simulink model "MotorFramework"  (R2026a)
settings: Solver=FixedStepAuto  StopTime=4  FixedStep=6.25e-5
undefined symbols (not defined in the file): McControl_Params, McRuntime_Init
settings Model: DataDictionary=McData.sldd  Creator=k  LastModifiedBy=k
settings OptimizationCC: UseDivisionForNetSlopeComputation=on  GainParamInheritBuiltInType=on  UseFloatMulNetSlope=on  InlineInvariantSignals=on  NoFixptDivByZeroProtection=on  EfficientFloat2IntCast=on  LifeSpan=1
settings RTWCC: SystemTargetFile=ert.tlc  GenerateReport=on  IncludeHyperlinkInReport=on  GenerateTraceInfo=on  GenerateTraceReport=on  GenerateTraceReportSl=on  GenerateTraceReportSf=on  GenerateTraceReportEml=on  GenerateCodeMetricsReport=on  Description=Embedded Coder
settings ERTTargetCC: GenerateSampleERTMain=on  IncludeMdlTerminateFcn=off  CombineSignalStateStructs=on  SupportComplex=off  SupportContinuousTime=on  SupportNonInlinedSFcns=on

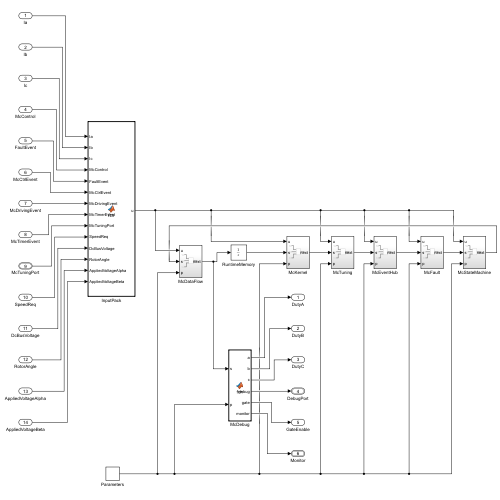
[thumbnail: Simulink's stored preview of the top-level diagram]
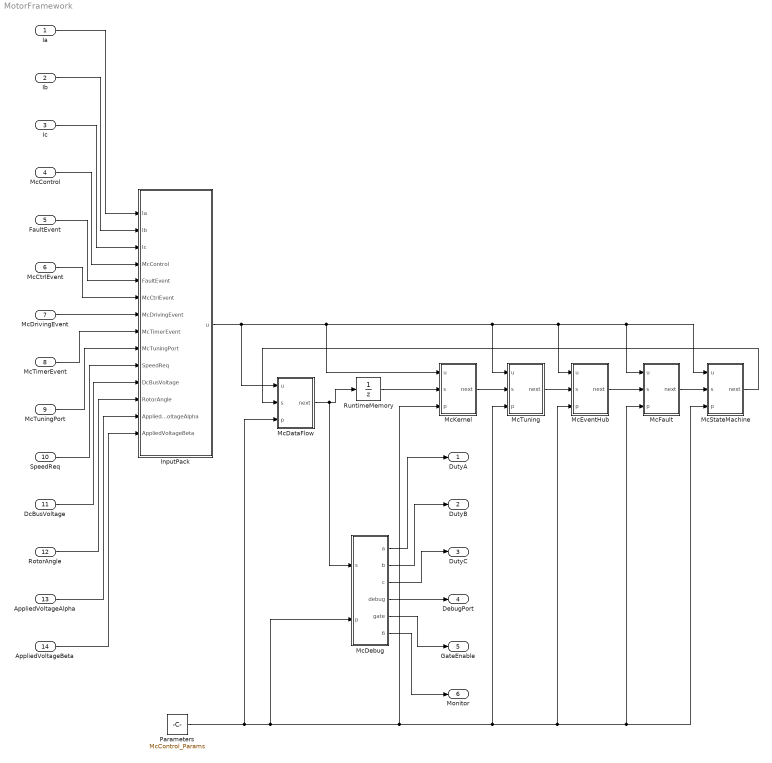
== system MotorFramework ==
  Ia : Inport  OutDataTypeStr=uint16  SampleTime=6.25e-5
  Ib : Inport  Port=2  OutDataTypeStr=uint16  SampleTime=6.25e-5
  Ic : Inport  Port=3  OutDataTypeStr=uint16  SampleTime=6.25e-5
  McControl : Inport  Port=4  OutDataTypeStr=uint8  SampleTime=6.25e-5
  FaultEvent : Inport  Port=5  OutDataTypeStr=boolean  SampleTime=6.25e-5
  McCtrlEvent : Inport  Port=6  OutDataTypeStr=boolean  SampleTime=6.25e-5
  McDrivingEvent : Inport  Port=7  OutDataTypeStr=boolean  SampleTime=6.25e-5
  McTimerEvent : Inport  Port=8  OutDataTypeStr=boolean  SampleTime=6.25e-5
  McTuningPort : Inport  Port=9  OutDataTypeStr=Bus: tMcTuning  SampleTime=6.25e-5
  SpeedReq : Inport  Port=10  OutDataTypeStr=single  SampleTime=6.25e-5
  DcBusVoltage : Inport  Port=11  OutDataTypeStr=single  SampleTime=6.25e-5
  RotorAngle : Inport  Port=12  OutDataTypeStr=single  SampleTime=6.25e-5
  AppliedVoltageAlpha : Inport  Port=13  OutDataTypeStr=single  SampleTime=6.25e-5
  AppliedVoltageBeta : Inport  Port=14  OutDataTypeStr=single  SampleTime=6.25e-5
  InputPack : MATLAB Function  TreatAsAtomicUnit=on
  McDataFlow : Subsystem
  McDebug : MATLAB Function  TreatAsAtomicUnit=on
  McEventHub : Subsystem
  McFault : Subsystem
  McKernel : Subsystem
  McStateMachine : Subsystem
  McTuning : Subsystem
  Parameters : Constant  Value=McControl_Params  OutDataTypeStr=Bus: tMcControlParams
  RuntimeMemory : UnitDelay  InitialCondition=McRuntime_Init  SampleTime=6.25e-5
  DutyA : Outport  OutDataTypeStr=uint16
  DutyB : Outport  Port=2  OutDataTypeStr=uint16
  DutyC : Outport  Port=3  OutDataTypeStr=uint16
  DebugPort : Outport  Port=4  OutDataTypeStr=Bus: tMcDebug
  GateEnable : Outport  Port=5  OutDataTypeStr=boolean
  Monitor : Outport  Port=6  OutDataTypeStr=Bus: tMcMonitor
  wires:
  Ia/1 -> InputPack/1(Ia)
  Ib/1 -> InputPack/2(Ib)
  Ic/1 -> InputPack/3(Ic)
  McControl/1 -> InputPack/4(McControl)
  FaultEvent/1 -> InputPack/5(FaultEvent)
  McCtrlEvent/1 -> InputPack/6(McCtrlEvent)
  McDrivingEvent/1 -> InputPack/7(McDrivingEvent)
  McTimerEvent/1 -> InputPack/8(McTimerEvent)
  McTuningPort/1 -> InputPack/9(McTuningPort)
  SpeedReq/1 -> InputPack/10(SpeedReq)
  DcBusVoltage/1 -> InputPack/11(DcBusVoltage)
  RotorAngle/1 -> InputPack/12(RotorAngle)
  AppliedVoltageAlpha/1 -> InputPack/13(AppliedVoltageAlpha)
  AppliedVoltageBeta/1 -> InputPack/14(AppliedVoltageBeta)
  InputPack/1(u) -> McStateMachine/1(u), McFault/1(u), McEventHub/1(u), McTuning/1(u), McKernel/1(u), McDataFlow/1(u)
  RuntimeMemory/1 -> McKernel/2(s)
  Parameters/1 -> McFault/3(p), McStateMachine/3(p), McEventHub/3(p), McTuning/3(p), McKernel/3(p), McDebug/2(p), McDataFlow/3(p)
  McKernel/1(next) -> McTuning/2(s)
  McTuning/1(next) -> McEventHub/2(s)
  McEventHub/1(next) -> McFault/2(s)
  McFault/1(next) -> McStateMachine/2(s)
  McStateMachine/1(next) -> McDataFlow/2(s)
  McDataFlow/1(next) -> RuntimeMemory/1, McDebug/1(s)
  McDebug/1(a) -> DutyA/1
  McDebug/2(b) -> DutyB/1
  McDebug/3(c) -> DutyC/1
  McDebug/4(debug) -> DebugPort/1
  McDebug/5(gate) -> GateEnable/1
  McDebug/6(monitor) -> Monitor/1

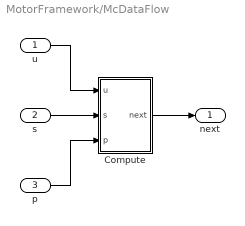
== system MotorFramework/McDataFlow ==
  u : Inport  OutDataTypeStr=Bus: tMcInput  SampleTime=6.25e-5
  s : Inport  Port=2  OutDataTypeStr=Bus: tMcRuntime  SampleTime=6.25e-5
  p : Inport  Port=3  OutDataTypeStr=Bus: tMcControlParams  SampleTime=6.25e-5
  Compute : MATLAB Function  TreatAsAtomicUnit=on
  next : Outport  OutDataTypeStr=Bus: tMcRuntime
  wires:
  Compute/1(next) -> next/1
  p/1 -> Compute/3(p)
  s/1 -> Compute/2(s)
  u/1 -> Compute/1(u)

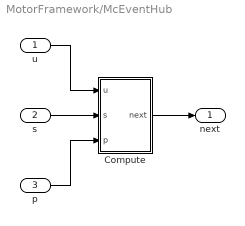
== system MotorFramework/McEventHub ==
  u : Inport  OutDataTypeStr=Bus: tMcInput  SampleTime=6.25e-5
  s : Inport  Port=2  OutDataTypeStr=Bus: tMcRuntime  SampleTime=6.25e-5
  p : Inport  Port=3  OutDataTypeStr=Bus: tMcControlParams  SampleTime=6.25e-5
  Compute : MATLAB Function  TreatAsAtomicUnit=on
  next : Outport  OutDataTypeStr=Bus: tMcRuntime
  wires:
  Compute/1(next) -> next/1
  p/1 -> Compute/3(p)
  s/1 -> Compute/2(s)
  u/1 -> Compute/1(u)

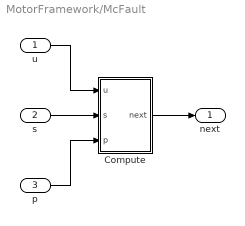
== system MotorFramework/McFault ==
  u : Inport  OutDataTypeStr=Bus: tMcInput  SampleTime=6.25e-5
  s : Inport  Port=2  OutDataTypeStr=Bus: tMcRuntime  SampleTime=6.25e-5
  p : Inport  Port=3  OutDataTypeStr=Bus: tMcControlParams  SampleTime=6.25e-5
  Compute : MATLAB Function  TreatAsAtomicUnit=on
  next : Outport  OutDataTypeStr=Bus: tMcRuntime
  wires:
  Compute/1(next) -> next/1
  p/1 -> Compute/3(p)
  s/1 -> Compute/2(s)
  u/1 -> Compute/1(u)

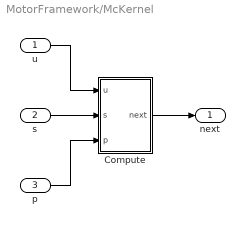
== system MotorFramework/McKernel ==
  u : Inport  OutDataTypeStr=Bus: tMcInput  SampleTime=6.25e-5
  s : Inport  Port=2  OutDataTypeStr=Bus: tMcRuntime  SampleTime=6.25e-5
  p : Inport  Port=3  OutDataTypeStr=Bus: tMcControlParams  SampleTime=6.25e-5
  Compute : MATLAB Function  TreatAsAtomicUnit=on
  next : Outport  OutDataTypeStr=Bus: tMcRuntime
  wires:
  Compute/1(next) -> next/1
  p/1 -> Compute/3(p)
  s/1 -> Compute/2(s)
  u/1 -> Compute/1(u)

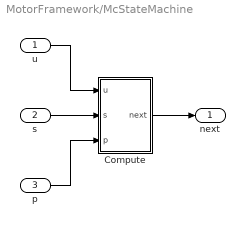
== system MotorFramework/McStateMachine ==
  u : Inport  OutDataTypeStr=Bus: tMcInput  SampleTime=6.25e-5
  s : Inport  Port=2  OutDataTypeStr=Bus: tMcRuntime  SampleTime=6.25e-5
  p : Inport  Port=3  OutDataTypeStr=Bus: tMcControlParams  SampleTime=6.25e-5
  Compute : MATLAB Function  TreatAsAtomicUnit=on
  next : Outport  OutDataTypeStr=Bus: tMcRuntime
  wires:
  Compute/1(next) -> next/1
  p/1 -> Compute/3(p)
  s/1 -> Compute/2(s)
  u/1 -> Compute/1(u)

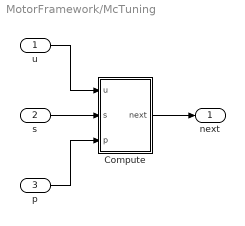
== system MotorFramework/McTuning ==
  u : Inport  OutDataTypeStr=Bus: tMcInput  SampleTime=6.25e-5
  s : Inport  Port=2  OutDataTypeStr=Bus: tMcRuntime  SampleTime=6.25e-5
  p : Inport  Port=3  OutDataTypeStr=Bus: tMcControlParams  SampleTime=6.25e-5
  Compute : MATLAB Function  TreatAsAtomicUnit=on
  next : Outport  OutDataTypeStr=Bus: tMcRuntime
  wires:
  Compute/1(next) -> next/1
  p/1 -> Compute/3(p)
  s/1 -> Compute/2(s)
  u/1 -> Compute/1(u)

== matlab function MotorFramework/McDebug ==
  data: s input; a output; p input; b output; c output; debug output Bus: tMcDebug; gate output; monitor output Bus: tMcMonitor
function [a,b,c,debug,gate,monitor]=fcn(s,p)
%#codegen
[counts,debug,monitor]=mc.monitor(s,p);
a=counts(1);b=counts(2);c=counts(3);gate=s.GateEnable;
end

== matlab function MotorFramework/InputPack ==
  data: Ia input; u output Bus: tMcInput; Ib input; Ic input; McControl input; FaultEvent input; McCtrlEvent input; McDrivingEvent input; McTimerEvent input; McTuningPort input; SpeedReq input; DcBusVoltage input; RotorAngle input; AppliedVoltageAlpha input; AppliedVoltageBeta input
function u=fcn(Ia,Ib,Ic,McControl,FaultEvent,McCtrlEvent,McDrivingEvent,McTimerEvent,McTuningPort,SpeedReq,DcBusVoltage,RotorAngle,AppliedVoltageAlpha,AppliedVoltageBeta)
%#codegen
u.CurrentRaw=[Ia;Ib;Ic];
u.Control=McControl;
u.Fault=FaultEvent;
u.CommandEvent=McCtrlEvent;
u.DrivingEvent=McDrivingEvent;
u.TimerEvent=McTimerEvent;
u.SpeedReq=SpeedReq;
u.Vdc=DcBusVoltage;
u.Position=RotorAngle;
u.AppliedVoltage=[AppliedVoltageAlpha;AppliedVoltageBeta];
u.Tuning=McTuningPort;
end

== matlab function MotorFramework/McKernel/Compute ==
  data: u input; next output Bus: tMcRuntime; s input; p input
function next=fcn(u,s,p)
%#codegen
next=mc.kernel(u,s,p);
end

== matlab function MotorFramework/McTuning/Compute ==
  data: u input; next output Bus: tMcRuntime; s input; p input
function next=fcn(u,s,p)
%#codegen
next=mc.tuning(u,s,p);
end

== matlab function MotorFramework/McEventHub/Compute ==
  data: u input; next output Bus: tMcRuntime; s input; p input
function next=fcn(u,s,p)
%#codegen
next=mc.event_hub(u,s,p);
end

== matlab function MotorFramework/McFault/Compute ==
  data: u input; next output Bus: tMcRuntime; s input; p input
function next=fcn(u,s,p)
%#codegen
next=mc.protection(u,s,p);
end

== matlab function MotorFramework/McStateMachine/Compute ==
  data: u input; next output Bus: tMcRuntime; s input; p input
function next=fcn(u,s,p)
%#codegen
next=mc.supervisor(u,s,p);
end

== matlab function MotorFramework/McDataFlow/Compute ==
  data: u input; next output Bus: tMcRuntime; s input; p input
function next=fcn(u,s,p)
%#codegen
next=mc.dataflow(u,s,p);
end
